simulink model "dsp_proj_v3_2024_n"  (R2025b)
settings: Solver=FixedStepDiscrete  StartTime=0.0  StopTime=1e-4  FixedStep=1/60e6  RelTol=1e-3
values from neighbouring files (symbols this model uses):
  b_1 = d_1.Coefficients    [fix.m]    (also in output.m; script_v2.m; stdmdl_2.m)
  b_2 = d_2.Coefficients    [fix.m]    (also in output.m; script_v2.m; stdmdl_2.m)
  b_3 = d_3.Coefficients    [fix.m]    (also in output.m; script_v2.m; stdmdl_2.m)
undefined symbols (not defined in the file or in its folder): dspblkCoreblockFVToolHelper, gcbh
libraries: hdlsllib x12, simulink x4
settings Model: Creator=UTSAB KARAN  LastModifiedBy=souma
settings SolverCC: AutoInsertRateTranBlk=on
settings OptimizationCC: BlockReduction=off  ConditionallyExecuteInputs=off
settings DebuggingCC: SingleTaskRateTransMsg=error

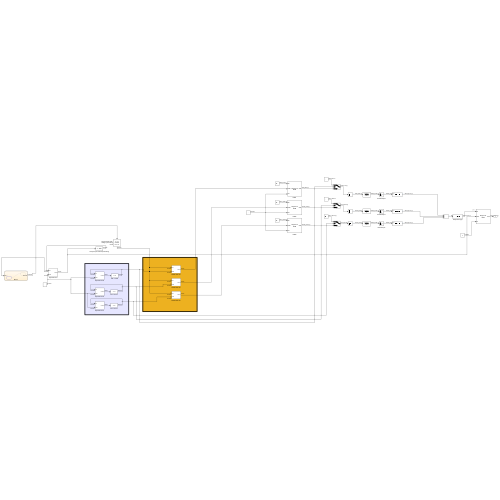
[thumbnail: Simulink's stored preview of the top-level diagram]
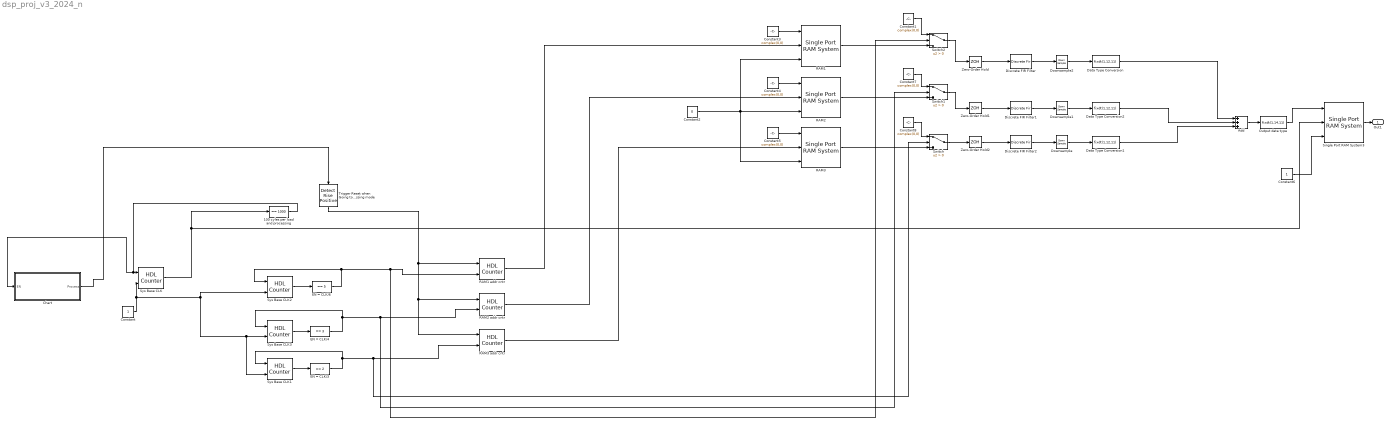
== system dsp_proj_v3_2024_n ==
  100 cyles per load and processing : simulink/Logic and Bit Operations/Compare To Constant  relop===  const=1000  OutDataTypeStr=boolean
  Add : Sum  Inputs=+++
  Chart : Stateflow chart  TreatAsAtomicUnit=on
  Constant : Constant  OutDataTypeStr=boolean
  Constant1 : Constant  Value=complex(0,0)  VectorParams1D=off  OutDataTypeStr=fixdt(1,8,6)  SampleTime=-1  LockScale=on
  Constant2 : Constant  Value=0  OutDataTypeStr=boolean
  Constant3 : Constant  Value=complex(0,0)  OutDataTypeStr=fixdt(1,8,6)
  Constant4 : Constant  Value=complex(0,0)  OutDataTypeStr=fixdt(1,10,8)
  Constant5 : Constant  Value=complex(0,0)  OutDataTypeStr=fixdt(1,12,10)
  Constant6 : Constant  OutDataTypeStr=boolean
  Constant7 : Constant  Value=complex(0,0)  VectorParams1D=off  OutDataTypeStr=fixdt(1,10,8)  SampleTime=-1  LockScale=on
  Constant8 : Constant  Value=complex(0,0)  VectorParams1D=off  OutDataTypeStr=fixdt(1,12,10)  SampleTime=-1  LockScale=on
  Data Type Conversion : DataTypeConversion  OutDataTypeStr=fixdt(1,12,11)  RndMeth=Floor
  Data Type Conversion1 : DataTypeConversion  OutDataTypeStr=fixdt(1,12,11)  RndMeth=Floor
  Data Type Conversion2 : DataTypeConversion  OutDataTypeStr=fixdt(1,12,11)  RndMeth=Floor
  Discrete FIR Filter : DiscreteFir  LoadFcn=dspblkCoreblockFVToolHelper(gcbh,'load');  FilterStructure=Direct form symmetric  Coefficients=b_1  CoefDataTypeStr=fixdt(1,25,24)
      settings: CopyFcn=dspblkCoreblockFVToolHelper(gcbh,'copy');  DeleteFcn=dspblkCoreblockFVToolHelper(gcbh,'close');  ModelCloseFcn=dspblkCoreblockFVToolHelper(gcbh,'close');  PreSaveFcn=dspblkCoreblockFVToolHelper(gcbh,'presave');  PostSaveFcn=dspblkCoreblockFVToolHelper(gcbh,'postsave');  CloseFcn=dspblkCoreblockFVToolHelper(gcbh,'close');
  Discrete FIR Filter1 : DiscreteFir  LoadFcn=dspblkCoreblockFVToolHelper(gcbh,'load');  FilterStructure=Direct form symmetric  Coefficients=b_2  CoefDataTypeStr=fixdt(1,25,24)
      settings: CopyFcn=dspblkCoreblockFVToolHelper(gcbh,'copy');  DeleteFcn=dspblkCoreblockFVToolHelper(gcbh,'close');  ModelCloseFcn=dspblkCoreblockFVToolHelper(gcbh,'close');  PreSaveFcn=dspblkCoreblockFVToolHelper(gcbh,'presave');  PostSaveFcn=dspblkCoreblockFVToolHelper(gcbh,'postsave');  CloseFcn=dspblkCoreblockFVToolHelper(gcbh,'close');
  Discrete FIR Filter2 : DiscreteFir  LoadFcn=dspblkCoreblockFVToolHelper(gcbh,'load');  FilterStructure=Direct form symmetric  Coefficients=b_3  CoefDataTypeStr=fixdt(1,25,24)
      settings: CopyFcn=dspblkCoreblockFVToolHelper(gcbh,'copy');  DeleteFcn=dspblkCoreblockFVToolHelper(gcbh,'close');  ModelCloseFcn=dspblkCoreblockFVToolHelper(gcbh,'close');  PreSaveFcn=dspblkCoreblockFVToolHelper(gcbh,'presave');  PostSaveFcn=dspblkCoreblockFVToolHelper(gcbh,'postsave');  CloseFcn=dspblkCoreblockFVToolHelper(gcbh,'close');
  Downsample : DownSample  N=5  RateOptions=Allow multirate processing
  Downsample1 : DownSample  N=5  RateOptions=Allow multirate processing
  Downsample2 : DownSample  N=5  RateOptions=Allow multirate processing
  EN = CLK/3 : simulink/Logic and Bit Operations/Compare To Constant  relop===  const=2  OutDataTypeStr=boolean
  EN = CLK/4 : simulink/Logic and Bit Operations/Compare To Constant  relop===  const=3  OutDataTypeStr=boolean
  EN = CLK/6 : simulink/Logic and Bit Operations/Compare To Constant  relop===  const=5  OutDataTypeStr=boolean
  Output data type : DataTypeConversion  OutDataTypeStr=fixdt(1,14,11)  SaturateOnIntegerOverflow=off  RndMeth=Floor  LockScale=on
  RAM1 : hdlsllib/HDL RAMs/Single Port RAM System  RAMType=Single port  AsyncRead=off  WriteOutputValue=New data  RAMInitialValue=ram1_init_data  allowBusInputs=off  WritesHaveOutput=on  NumReads=0  NumWrites=1  SimulateUsing=Code generation  ModelRAMDelay=on  VectorAccess=Parallel
  RAM1 addr cntr : hdlsllib/Sources/HDL Counter  CountType=Count limited  CountInit=0  CountStep=1  CountMax=3000  CountFromType=Initial value  CountFrom=0  CountResetPort=on  CountLoadPort=off  CountEnbPort=on  CountDirPort=off  CountHitOutputPort=off  CountDataType=Unsigned  CountWordLen=12  CountFracLen=0  CountSampTime=1
  RAM2 : hdlsllib/HDL RAMs/Single Port RAM System  RAMType=Single port  AsyncRead=off  WriteOutputValue=New data  RAMInitialValue=ram2_init_data  allowBusInputs=off  WritesHaveOutput=on  NumReads=0  NumWrites=1  SimulateUsing=Code generation  ModelRAMDelay=on  VectorAccess=Parallel
  RAM2 addr cntr : hdlsllib/Sources/HDL Counter  CountType=Count limited  CountInit=0  CountStep=1  CountMax=3000  CountFromType=Initial value  CountFrom=0  CountResetPort=on  CountLoadPort=off  CountEnbPort=on  CountDirPort=off  CountHitOutputPort=off  CountDataType=Unsigned  CountWordLen=12  CountFracLen=0  CountSampTime=1
  RAM3 : hdlsllib/HDL RAMs/Single Port RAM System  RAMType=Single port  AsyncRead=off  WriteOutputValue=New data  RAMInitialValue=ram3_init_data  allowBusInputs=off  WritesHaveOutput=on  NumReads=0  NumWrites=1  SimulateUsing=Code generation  ModelRAMDelay=on  VectorAccess=Parallel
  RAM3 addr cntr : hdlsllib/Sources/HDL Counter  CountType=Count limited  CountInit=0  CountStep=1  CountMax=3000  CountFromType=Initial value  CountFrom=0  CountResetPort=on  CountLoadPort=off  CountEnbPort=on  CountDirPort=off  CountHitOutputPort=off  CountDataType=Unsigned  CountWordLen=12  CountFracLen=0  CountSampTime=1
  Single Port RAM System3 : hdlsllib/HDL RAMs/Single Port RAM System  RAMType=Single port  AsyncRead=off  WriteOutputValue=New data  RAMInitialValue=0  allowBusInputs=off  WritesHaveOutput=on  NumReads=0  NumWrites=1  SimulateUsing=Code generation  ModelRAMDelay=on  VectorAccess=Parallel
  Switch : Switch  Criteria=u2 > Threshold  SaturateOnIntegerOverflow=off  InputSameDT=off
  Switch1 : Switch  Criteria=u2 > Threshold  SaturateOnIntegerOverflow=off  InputSameDT=off
  Switch2 : Switch  Criteria=u2 > Threshold  SaturateOnIntegerOverflow=off  InputSameDT=off
  Sys Base CLK : hdlsllib/Sources/HDL Counter  CountType=Count limited  CountInit=0  CountStep=1  CountMax=1000  CountFromType=Initial value  CountFrom=0  CountResetPort=on  CountLoadPort=off  CountEnbPort=on  CountDirPort=off  CountHitOutputPort=off  CountDataType=Unsigned  CountWordLen=12  CountFracLen=0  CountSampTime=1
  Sys Base CLK1 : hdlsllib/Sources/HDL Counter  CountType=Count limited  CountInit=0  CountStep=1  CountMax=2  CountFromType=Initial value  CountFrom=0  CountResetPort=on  CountLoadPort=off  CountEnbPort=on  CountDirPort=off  CountHitOutputPort=off  CountDataType=Unsigned  CountWordLen=12  CountFracLen=0  CountSampTime=1
  Sys Base CLK2 : hdlsllib/Sources/HDL Counter  CountType=Count limited  CountInit=0  CountStep=1  CountMax=5  CountFromType=Initial value  CountFrom=0  CountResetPort=on  CountLoadPort=off  CountEnbPort=on  CountDirPort=off  CountHitOutputPort=off  CountDataType=Unsigned  CountWordLen=12  CountFracLen=0  CountSampTime=1
  Sys Base CLK3 : hdlsllib/Sources/HDL Counter  CountType=Count limited  CountInit=0  CountStep=1  CountMax=3  CountFromType=Initial value  CountFrom=0  CountResetPort=on  CountLoadPort=off  CountEnbPort=on  CountDirPort=off  CountHitOutputPort=off  CountDataType=Unsigned  CountWordLen=12  CountFracLen=0  CountSampTime=1
  Trigger Reset when Going to processing mode : hdlsllib/Logic and Bit Operations/Detect Rise Positive  vinit=0  OutDataTypeStr=boolean
  Zero-Order Hold : ZeroOrderHold  SampleTime=1/60e6
  Zero-Order Hold1 : ZeroOrderHold  SampleTime=1/60e6
  Zero-Order Hold2 : ZeroOrderHold  SampleTime=1/60e6
  Out1 : Outport
  wires:
  Sys Base CLK/1 -> Single Port RAM System3/2, 100 cyles per load and processing/1
  Constant/1 -> Sys Base CLK3/2, Sys Base CLK1/2, Sys Base CLK2/2, Sys Base CLK/2
  100 cyles per load and processing/1 -> Chart/1(EN), Sys Base CLK/1
  EN = CLK/3/1 -> Sys Base CLK1/1, RAM3 addr cntr/2, Switch/2
  Switch1/1 -> Zero-Order Hold1/1
  Add/1 -> Output data type/1
  Output data type/1 -> Single Port RAM System3/1
  Chart/1(Process) -> Trigger Reset when Going to processing mode/1
  Trigger Reset when Going to processing mode/1 -> RAM1 addr cntr/1, RAM3 addr cntr/1, RAM2 addr cntr/1
  RAM1/1 -> Switch2/3
  RAM1 addr cntr/1 -> RAM1/2
  RAM2 addr cntr/1 -> RAM2/2
  Sys Base CLK1/1 -> EN = CLK/3/1
  Sys Base CLK2/1 -> EN = CLK/6/1
  EN = CLK/4/1 -> Sys Base CLK3/1, RAM2 addr cntr/2, Switch1/2
  Sys Base CLK3/1 -> EN = CLK/4/1
  RAM3 addr cntr/1 -> RAM3/2
  Constant2/1 -> RAM1/3, RAM2/3, RAM3/3
  EN = CLK/6/1 -> RAM1 addr cntr/2, Switch2/2, Sys Base CLK2/1
  RAM2/1 -> Switch1/3
  RAM3/1 -> Switch/3
  Switch/1 -> Zero-Order Hold2/1
  Switch2/1 -> Zero-Order Hold/1
  Discrete FIR Filter/1 -> Downsample2/1
  Discrete FIR Filter1/1 -> Downsample1/1
  Discrete FIR Filter2/1 -> Downsample/1
  Zero-Order Hold/1 -> Discrete FIR Filter/1
  Zero-Order Hold1/1 -> Discrete FIR Filter1/1
  Zero-Order Hold2/1 -> Discrete FIR Filter2/1
  Downsample2/1 -> Data Type Conversion/1
  Downsample1/1 -> Data Type Conversion2/1
  Downsample/1 -> Data Type Conversion1/1
  Data Type Conversion1/1 -> Add/3
  Data Type Conversion2/1 -> Add/2
  Data Type Conversion/1 -> Add/1
  Constant5/1 -> RAM3/1
  Constant4/1 -> RAM2/1
  Constant3/1 -> RAM1/1
  Constant6/1 -> Single Port RAM System3/3
  Constant1/1 -> Switch2/1
  Constant7/1 -> Switch1/1
  Constant8/1 -> Switch/1
  Single Port RAM System3/1 -> Out1/1

== stateflow chart dsp_proj_v3_2024_n/Chart ==
  settings: stateMachineType=MOORE_MACHINE  executeAtInitialization=1
  state Processing
    Process = true
  state Data_Loading
    Process = false
  Data_Loading -> Processing : [ EN==1]
  (default) -> Data_Loading
  data: Process output; EN input
